simulink model "e5_3blocks_nn"  (R2020a)
settings: Solver=VariableStepAuto  StartTime=0.0  StopTime=10.0  RelTol=1e-3
undefined symbols (not defined in the file or in its folder): Quad
libraries: neural x123
(part 1 of 6)
settings Model: Creator=kekatos  LastModifiedBy=kekatos

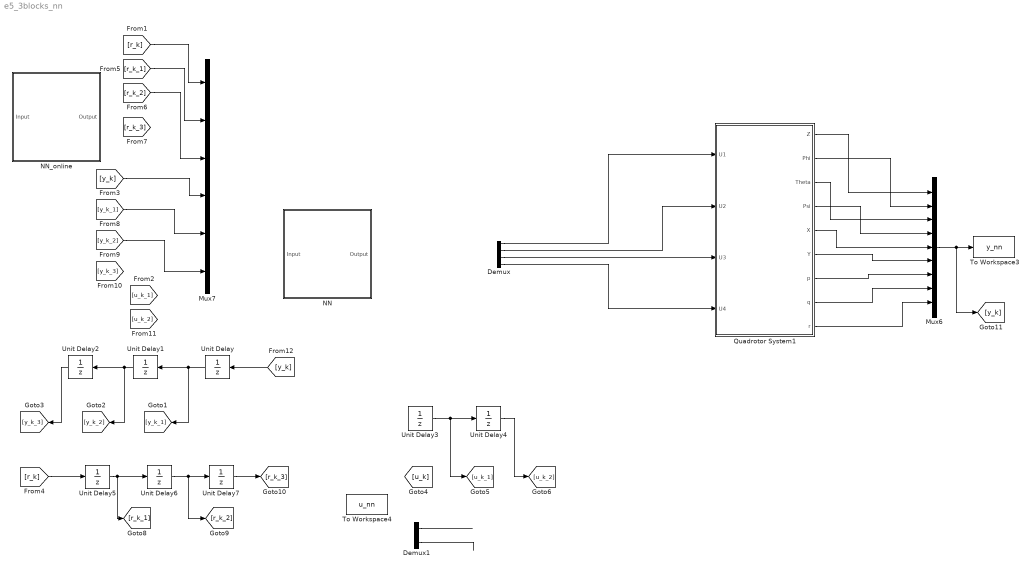
== system e5_3blocks_nn ==
  Demux : Demux
  Demux1 : Demux  Outputs=2
  Mux6 : Mux  Inputs=9
  Mux7 : Mux  Inputs=6
  NN : Subsystem
      mask help: Feed-Forward Neural Network
      mask Display: e = 0.06;c1 = [120 150 230]/255;c2 = ([120 150 230]+0)/383;c3 = ([120 150 230]+128)/383;patch([0 1 1 0],[0 0 1 1],c1);patch([0 1 1 1-e 1-e 0+e],[0 0 1 1-e 0+e 0+e],c2);patch([0 0 1 1-e 0+e 0+e],[0 1 1 1-e 1-e 0+e],c3);plot([0 1 1 0 0],[0 0 1 1 0]);fprintf('NNET');port_label('input',1,' Input');port_label('output',1,'Output ');
  NN_online : Subsystem
      mask help: Feed-Forward Neural Network
      mask Display: e = 0.06;c1 = [120 150 230]/255;c2 = ([120 150 230]+0)/383;c3 = ([120 150 230]+128)/383;patch([0 1 1 0],[0 0 1 1],c1);patch([0 1 1 1-e 1-e 0+e],[0 0 1 1-e 0+e 0+e],c2);patch([0 0 1 1-e 0+e 0+e],[0 1 1 1-e 1-e 0+e],c3);plot([0 1 1 0 0],[0 0 1 1 0]);fprintf('NNET');port_label('input',1,' Input');port_label('output',1,'Output ');
  Quadrotor System1 : Subsystem
  To Workspace3 : ToWorkspace  VariableName=y_nn  SaveFormat=Structure With Time  SampleTime=0.01
  To Workspace4 : ToWorkspace  VariableName=u_nn  SaveFormat=Structure With Time  SampleTime=0.01
  Unit Delay{,1..7} (8 alike) : UnitDelay  SampleTime=-1  HasFrameUpgradeWarning=on
  wires:
  Quadrotor System1/7(p) -> Mux6/7
  Unit Delay2/1 -> [y_k_3]
  Quadrotor System1/1(Z) -> Mux6/1
  [y_k] -> Unit Delay/1
  Unit Delay6/1 -> [r_k_2], Unit Delay7/1
  [r_k] -> Mux7/1
  Quadrotor System1/4(Psi) -> Mux6/4
  Unit Delay4/1 -> [u_k_2]
  Quadrotor System1/9(r) -> Mux6/9
  Unit Delay7/1 -> [r_k_3]
  Unit Delay1/1 -> Unit Delay2/1, [y_k_2]
  Unit Delay/1 -> Unit Delay1/1, [y_k_1]
  [r_k_2] -> Mux7/3
  Quadrotor System1/5(X) -> Mux6/5
  Demux/1 -> Quadrotor System1/1(U1)
  Mux6/1 -> [y_k], To Workspace3/1
  Unit Delay3/1 -> [u_k_1], Unit Delay4/1
  Quadrotor System1/3(Theta) -> Mux6/3
  Demux1/1 -> ?
  Quadrotor System1/8(q) -> Mux6/8
  [y_k] -> Mux7/4
  Demux/4 -> Quadrotor System1/4(U4)
  Quadrotor System1/2(Phi) -> Mux6/2
  Demux1/2 -> ?
  Quadrotor System1/6(Y) -> Mux6/6
  Demux/2 -> Quadrotor System1/2(U2)
  [y_k_2] -> Mux7/6
  [r_k_1] -> Mux7/2
  [y_k_1] -> Mux7/5
  Demux/3 -> Quadrotor System1/3(U3)
  [r_k] -> Unit Delay5/1
  Unit Delay5/1 -> [r_k_1], Unit Delay6/1

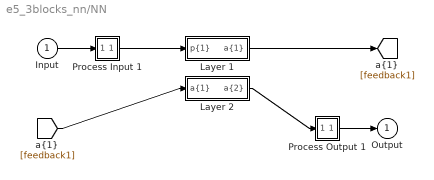
== system e5_3blocks_nn/NN ==
  Input : Inport  PortDimensions=15
      mask Display: e = 0.06;c1 = [120 230 180]/255;c2 = ([120 230 180]+0)/(256+128);c3 = ([120 230 180]+128)/(256+128);patch([0 1 1 0],[0 0 1 1],c1);patch([0 1 1 1-e 1-e 0+e],[0 0 1 1-e 0+e 0+e],c2);patch([0 0 1 1-e 0+e 0+e],[0 1 1 1-e 1-e 0+e],c3);plot([0 1 1 0 0],[0 0 1 1 0]);
  Layer 1 : Subsystem
      mask Display: e = 0.06;c1 = [120 150 230]/255;c2 = ([120 150 230]+0)/383;c3 = ([120 150 230]+128)/383;patch([0 1 1 0],[0 0 1 1],c1);patch([0 1 1 1-e 1-e 0+e],[0 0 1 1-e 0+e 0+e],c2);patch([0 0 1 1-e 0+e 0+e],[0 1 1 1-e 1-e 0+e],c3);plot([0 1 1 0 0],[0 0 1 1 0]);
  Layer 2 : Subsystem
      mask Display: e = 0.06;c1 = [120 150 230]/255;c2 = ([120 150 230]+0)/383;c3 = ([120 150 230]+128)/383;patch([0 1 1 0],[0 0 1 1],c1);patch([0 1 1 1-e 1-e 0+e],[0 0 1 1-e 0+e 0+e],c2);patch([0 0 1 1-e 0+e 0+e],[0 1 1 1-e 1-e 0+e],c3);plot([0 1 1 0 0],[0 0 1 1 0]);
  Process Input 1 : Subsystem
      mask Display: e = 0.06;c1 = [120 150 230]/255;c2 = ([120 150 230]+0)/383;c3 = ([120 150 230]+128)/383;patch([0 1 1 0],[0 0 1 1],c1);patch([0 1 1 1-e 1-e 0+e],[0 0 1 1-e 0+e 0+e],c2);patch([0 0 1 1-e 0+e 0+e],[0 1 1 1-e 1-e 0+e],c3);plot([0 1 1 0 0],[0 0 1 1 0]);
  Process Output 1 : Subsystem
      mask Display: e = 0.06;c1 = [120 150 230]/255;c2 = ([120 150 230]+0)/383;c3 = ([120 150 230]+128)/383;patch([0 1 1 0],[0 0 1 1],c1);patch([0 1 1 1-e 1-e 0+e],[0 0 1 1-e 0+e 0+e],c2);patch([0 0 1 1-e 0+e 0+e],[0 1 1 1-e 1-e 0+e],c3);plot([0 1 1 0 0],[0 0 1 1 0]);
  Output : Outport  InitialOutput=[0;0]
      mask Display: e = 0.06;c1 = [120 230 180]/255;c2 = ([120 230 180]+0)/(256+128);c3 = ([120 230 180]+128)/(256+128);patch([0 1 1 0],[0 0 1 1],c1);patch([0 1 1 1-e 1-e 0+e],[0 0 1 1-e 0+e 0+e],c2);patch([0 0 1 1-e 0+e 0+e],[0 1 1 1-e 1-e 0+e],c3);plot([0 1 1 0 0],[0 0 1 1 0]);
  wires:
  Input/1 -> Process Input 1/1(x)
  Process Output 1/1(y) -> Output/1
  Process Input 1/1(p) -> Layer 1/1("p{1}")
  Layer 1/1("a{1}") -> [feedback1]
  [feedback1] -> Layer 2/1("a{1} ")
  Layer 2/1("a{2}") -> Process Output 1/1(a)

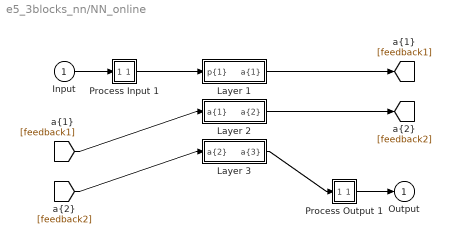
== system e5_3blocks_nn/NN_online ==
  Input : Inport  PortDimensions=20
      mask Display: e = 0.06;c1 = [120 230 180]/255;c2 = ([120 230 180]+0)/(256+128);c3 = ([120 230 180]+128)/(256+128);patch([0 1 1 0],[0 0 1 1],c1);patch([0 1 1 1-e 1-e 0+e],[0 0 1 1-e 0+e 0+e],c2);patch([0 0 1 1-e 0+e 0+e],[0 1 1 1-e 1-e 0+e],c3);plot([0 1 1 0 0],[0 0 1 1 0]);
  Layer 1 : Subsystem
      mask Display: e = 0.06;c1 = [120 150 230]/255;c2 = ([120 150 230]+0)/383;c3 = ([120 150 230]+128)/383;patch([0 1 1 0],[0 0 1 1],c1);patch([0 1 1 1-e 1-e 0+e],[0 0 1 1-e 0+e 0+e],c2);patch([0 0 1 1-e 0+e 0+e],[0 1 1 1-e 1-e 0+e],c3);plot([0 1 1 0 0],[0 0 1 1 0]);
  Layer 2 : Subsystem
      mask Display: e = 0.06;c1 = [120 150 230]/255;c2 = ([120 150 230]+0)/383;c3 = ([120 150 230]+128)/383;patch([0 1 1 0],[0 0 1 1],c1);patch([0 1 1 1-e 1-e 0+e],[0 0 1 1-e 0+e 0+e],c2);patch([0 0 1 1-e 0+e 0+e],[0 1 1 1-e 1-e 0+e],c3);plot([0 1 1 0 0],[0 0 1 1 0]);
  Layer 3 : Subsystem
      mask Display: e = 0.06;c1 = [120 150 230]/255;c2 = ([120 150 230]+0)/383;c3 = ([120 150 230]+128)/383;patch([0 1 1 0],[0 0 1 1],c1);patch([0 1 1 1-e 1-e 0+e],[0 0 1 1-e 0+e 0+e],c2);patch([0 0 1 1-e 0+e 0+e],[0 1 1 1-e 1-e 0+e],c3);plot([0 1 1 0 0],[0 0 1 1 0]);
  Process Input 1 : Subsystem
      mask Display: e = 0.06;c1 = [120 150 230]/255;c2 = ([120 150 230]+0)/383;c3 = ([120 150 230]+128)/383;patch([0 1 1 0],[0 0 1 1],c1);patch([0 1 1 1-e 1-e 0+e],[0 0 1 1-e 0+e 0+e],c2);patch([0 0 1 1-e 0+e 0+e],[0 1 1 1-e 1-e 0+e],c3);plot([0 1 1 0 0],[0 0 1 1 0]);
  Process Output 1 : Subsystem
      mask Display: e = 0.06;c1 = [120 150 230]/255;c2 = ([120 150 230]+0)/383;c3 = ([120 150 230]+128)/383;patch([0 1 1 0],[0 0 1 1],c1);patch([0 1 1 1-e 1-e 0+e],[0 0 1 1-e 0+e 0+e],c2);patch([0 0 1 1-e 0+e 0+e],[0 1 1 1-e 1-e 0+e],c3);plot([0 1 1 0 0],[0 0 1 1 0]);
  Output : Outport  InitialOutput=[0;0]
      mask Display: e = 0.06;c1 = [120 230 180]/255;c2 = ([120 230 180]+0)/(256+128);c3 = ([120 230 180]+128)/(256+128);patch([0 1 1 0],[0 0 1 1],c1);patch([0 1 1 1-e 1-e 0+e],[0 0 1 1-e 0+e 0+e],c2);patch([0 0 1 1-e 0+e 0+e],[0 1 1 1-e 1-e 0+e],c3);plot([0 1 1 0 0],[0 0 1 1 0]);
  wires:
  Input/1 -> Process Input 1/1(x)
  Process Output 1/1(y) -> Output/1
  Process Input 1/1(p) -> Layer 1/1("p{1}")
  Layer 1/1("a{1}") -> [feedback1]
  [feedback1] -> Layer 2/1("a{1} ")
  Layer 2/1("a{2}") -> [feedback2]
  [feedback2] -> Layer 3/1("a{2} ")
  Layer 3/1("a{3}") -> Process Output 1/1(a)

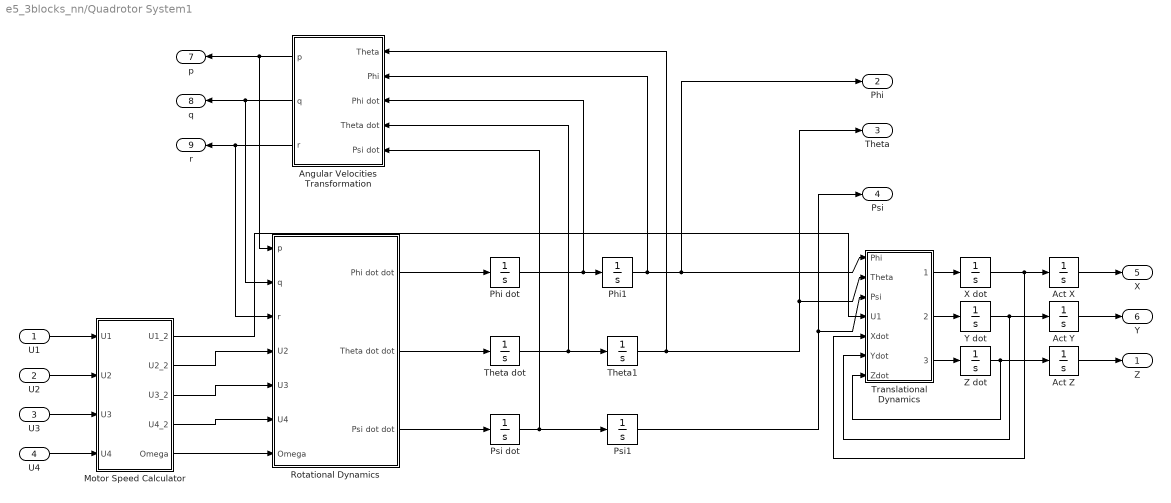
== system e5_3blocks_nn/Quadrotor System1 ==
  U1 : Inport
  U2 : Inport  Port=2
  U3 : Inport  Port=3
  U4 : Inport  Port=4
  Act X : Integrator
  Act Y : Integrator
  Act Z : Integrator
  Angular Velocities Transformation : Subsystem
  Motor Speed Calculator : Subsystem
  Phi dot : Integrator
  Phi1 : Integrator  ZeroCross=off
  Psi dot : Integrator  ZeroCross=off
  Psi1 : Integrator  ZeroCross=off
  Rotational Dynamics : Subsystem
  Theta dot : Integrator  ZeroCross=off
  Theta1 : Integrator  ZeroCross=off
  Translational Dynamics : Subsystem
  X dot : Integrator
  Y dot : Integrator
  Z dot : Integrator
  Z : Outport  VectorParamsAs1DForOutWhenUnconnected=off
  Phi : Outport  Port=2  VectorParamsAs1DForOutWhenUnconnected=off
  Theta : Outport  Port=3  VectorParamsAs1DForOutWhenUnconnected=off
  Psi : Outport  Port=4  VectorParamsAs1DForOutWhenUnconnected=off
  X : Outport  Port=5  VectorParamsAs1DForOutWhenUnconnected=off
  Y : Outport  Port=6  VectorParamsAs1DForOutWhenUnconnected=off
  p : Outport  Port=7  VectorParamsAs1DForOutWhenUnconnected=off
  q : Outport  Port=8  VectorParamsAs1DForOutWhenUnconnected=off
  r : Outport  Port=9  VectorParamsAs1DForOutWhenUnconnected=off
  wires:
  Rotational Dynamics/2(Theta dot dot) -> Theta dot/1
  Motor Speed Calculator/5(Omega) -> Rotational Dynamics/7(Omega)
  Phi1/1 -> Translational Dynamics/1(Phi), Phi/1, Angular Velocities Transformation/2(Phi)
  Theta1/1 -> Translational Dynamics/2(Theta), Theta/1, Angular Velocities Transformation/1(Theta)
  Psi1/1 -> Translational Dynamics/3(Psi), Psi/1
  Translational Dynamics/1(x dotdot) -> X dot/1
  X dot/1 -> Act X/1, Translational Dynamics/5(Xdot)
  Y dot/1 -> Act Y/1, Translational Dynamics/6(Ydot)
  Translational Dynamics/2(y dotdot) -> Y dot/1
  Z dot/1 -> Translational Dynamics/7(Zdot), Act Z/1
  Translational Dynamics/3(z dotdot) -> Z dot/1
  Act X/1 -> X/1
  Act Y/1 -> Y/1
  Act Z/1 -> Z/1
  Psi dot/1 -> Psi1/1, Angular Velocities Transformation/5(Psi dot)
  Theta dot/1 -> Theta1/1, Angular Velocities Transformation/4(Theta dot)
  Phi dot/1 -> Phi1/1, Angular Velocities Transformation/3(Phi dot)
  Rotational Dynamics/3(Psi dot dot) -> Psi dot/1
  Rotational Dynamics/1(Phi dot dot) -> Phi dot/1
  U4/1 -> Motor Speed Calculator/4(U4)
  U2/1 -> Motor Speed Calculator/2(U2)
  U3/1 -> Motor Speed Calculator/3(U3)
  Motor Speed Calculator/2(U2_2) -> Rotational Dynamics/4(U2)
  Motor Speed Calculator/3(U3_2) -> Rotational Dynamics/5(U3)
  Motor Speed Calculator/1(U1_2) -> Translational Dynamics/4(U1)
  Motor Speed Calculator/4(U4_2) -> Rotational Dynamics/6(U4)
  Angular Velocities Transformation/1(p) -> Rotational Dynamics/1(p), p/1
  Angular Velocities Transformation/2(q) -> Rotational Dynamics/2(q), q/1
  Angular Velocities Transformation/3(r) -> Rotational Dynamics/3(r), r/1
  U1/1 -> Motor Speed Calculator/1(U1)

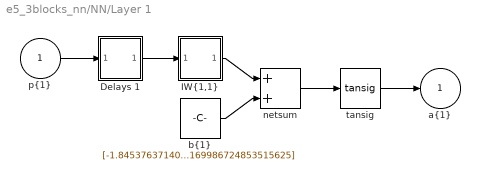
== system e5_3blocks_nn/NN/Layer 1 ==
  "p{1}" : Inport  PortDimensions=15
      mask Display: e = 0.06;c1 = [120 230 180]/255;c2 = ([120 230 180]+0)/(256+128);c3 = ([120 230 180]+128)/(256+128);patch([0 1 1 0],[0 0 1 1],c1);patch([0 1 1 1-e 1-e 0+e],[0 0 1 1-e 0+e 0+e],c2);patch([0 0 1 1-e 0+e 0+e],[0 1 1 1-e 1-e 0+e],c3);plot([0 1 1 0 0],[0 0 1 1 0]);
  Delays 1 : Subsystem
      mask Display: e = 0.06;c1 = [120 150 230]/255;c2 = ([120 150 230]+0)/383;c3 = ([120 150 230]+128)/383;patch([0 1 1 0],[0 0 1 1],c1);patch([0 1 1 1-e 1-e 0+e],[0 0 1 1-e 0+e 0+e],c2);patch([0 0 1 1-e 0+e 0+e],[0 1 1 1-e 1-e 0+e],c3);plot([0 1 1 0 0],[0 0 1 1 0]);disp('0');
  "IW{1,1}" : Subsystem
      mask Display: e = 0.06;c1 = [120 150 230]/255;c2 = ([120 150 230]+0)/383;c3 = ([120 150 230]+128)/383;patch([0 1 1 0],[0 0 1 1],c1);patch([0 1 1 1-e 1-e 0+e],[0 0 1 1-e 0+e 0+e],c2);patch([0 0 1 1-e 0+e 0+e],[0 1 1 1-e 1-e 0+e],c3);plot([0 1 1 0 0],[0 0 1 1 0]);disp('W');
  "b{1}" : Constant  Value=[-1.84537637140731280993577456683851778507232666015625;-1.7532825244992047419856362466816790401935577392578125;1.71407838156578673505237020435743033885955810546875;-1.6342052333083547654979383878526277840137481689453125;-1.5438537489742396591196893496089614927768707275390625;1.4283080018807214894849266784149222075939178466796875;-1.404821018307291780047307838685810565948486328125;1.287885767879537457503147379611618816852569580078125;1.25502611674529962471069666207768023014068603515625;1.0972360429977421336644738403265364468097686767578125;1.131430962279293073180497231078334152698516845703125;-0.9955530066140656497708505412447266280651092529296875;-0.89412837469389450095746951774344779551029205322265625;0.85010871782267416474354604360996745526790618896484375;-0.80545016544390790613761055283248424530029296875;-0.70922638754411959638446205644868314266204833984375;-0.63105719893839429257553774732514284551143646240234375;-0.569988447775239048809226005687378346920013427734375;0.477593047053590902262243389486684463918209075927734375;0.403175590821758189630230617694905959069728851318359375;0.358673720801043760531001680647023022174835205078125;-0.2482304075266782150688271713079302571713924407958984375;0.15068110824116487389545682162861339747905731201171875;-0.1602803495511306020038233555169426836073398590087890625;-0.0987868360797714839538485875891637988388538360595703125;0.04171171965434290751506551941929501481354236602783203125;0.0939112815207025775077198659346322529017925262451171875;-0.177186006071735346889539641779265366494655609130859375;0.2396368639811528866712109220316051505506038665771484375;0.342981184701568242445546275121159851551055908203125;0.416928111920932209510937127561192028224468231201171875;-0.495950560740119616998100582350161857903003692626953125;-0.590456977511941705216713671688921749591827392578125;-0.6649151320152437705246484256349503993988037109375;-0.608626845880423150703109058667905628681182861328125;0.79801769557657376008563687719288282096385955810546875;0.89966865010810692648846043084631673991680145263671875;0.9564815597009614922541231862851418554782867431640625;-1.04442351552266732284124373109079897403717041015625;-1.0713399950107189706471899626194499433040618896484375;-1.191236975152814903111675448599271476268768310546875;-1.1699716443134151599991810144274495542049407958984375;-1.29708105375885995869111866340972483158111572265625;1.3771740284091971151525513050728477537631988525390625;1.3780962923269959308214538395986892282962799072265625;1.53107763486454206969256119919009506702423095703125;-1.625607738312811800795998351532034575939178466796875;-1.698033535260649262710330731351859867572784423828125;-1.740593156442128641714361947379074990749359130859375;-1.7825772239617221348595421659410931169986724853515625]
      mask Display: e = 0.06;c1 = [120 150 230]/255;c2 = ([120 150 230]+0)/383;c3 = ([120 150 230]+128)/383;patch([0 1 1 0],[0 0 1 1],c1);patch([0 1 1 1-e 1-e 0+e],[0 0 1 1-e 0+e 0+e],c2);patch([0 0 1 1-e 0+e 0+e],[0 1 1 1-e 1-e 0+e],c3);plot([0 1 1 0 0],[0 0 1 1 0]);disp('b');
  netsum : Sum  Inputs=2  InputSameDT=on  SaturateOnIntegerOverflow=on  OutDataTypeStr=Inherit: Same as first input
      mask Display: e = 0.06;c1 = [120 150 230]/255;c2 = ([120 150 230]+0)/383;c3 = ([120 150 230]+128)/383;patch([0 1 1 0],[0 0 1 1],c1);patch([0 1 1 1-e 1-e 0+e],[0 0 1 1-e 0+e 0+e],c2);patch([0 0 1 1-e 0+e 0+e],[0 1 1 1-e 1-e 0+e],c3);plot([0 1 1 0 0],[0 0 1 1 0]);disp('+');
  tansig : neural/Transfer Functions/tansig
  "a{1}" : Outport  InitialOutput=[0;0;0;0;0;0;0;0;0;0;0;0;0;0;0;0;0;0;0;0;0;0;0;0;0;0;0;0;0;0;0;0;0;0;0;0;0;0;0;0;0;0;0;0;0;0;0;0;0;0]
      mask Display: e = 0.06;c1 = [120 230 180]/255;c2 = ([120 230 180]+0)/(256+128);c3 = ([120 230 180]+128)/(256+128);patch([0 1 1 0],[0 0 1 1],c1);patch([0 1 1 1-e 1-e 0+e],[0 0 1 1-e 0+e 0+e],c2);patch([0 0 1 1-e 0+e 0+e],[0 1 1 1-e 1-e 0+e],c3);plot([0 1 1 0 0],[0 0 1 1 0]);
  wires:
  "p{1}"/1 -> Delays 1/1("p{1}")
  Delays 1/1("pd{1,1}") -> "IW{1,1}"/1("pd{1,1}")
  "IW{1,1}"/1("iz{1,1}") -> netsum/1
  "b{1}"/1 -> netsum/2
  netsum/1 -> tansig/1
  tansig/1 -> "a{1}"/1

== system e5_3blocks_nn/NN/Layer 2 ==
  "a{1} " : Inport  PortDimensions=50
      mask Display: e = 0.06;c1 = [120 230 180]/255;c2 = ([120 230 180]+0)/(256+128);c3 = ([120 230 180]+128)/(256+128);patch([0 1 1 0],[0 0 1 1],c1);patch([0 1 1 1-e 1-e 0+e],[0 0 1 1-e 0+e 0+e],c2);patch([0 0 1 1-e 0+e 0+e],[0 1 1 1-e 1-e 0+e],c3);plot([0 1 1 0 0],[0 0 1 1 0]);
  Delays 1 : Subsystem
      mask Display: e = 0.06;c1 = [120 150 230]/255;c2 = ([120 150 230]+0)/383;c3 = ([120 150 230]+128)/383;patch([0 1 1 0],[0 0 1 1],c1);patch([0 1 1 1-e 1-e 0+e],[0 0 1 1-e 0+e 0+e],c2);patch([0 0 1 1-e 0+e 0+e],[0 1 1 1-e 1-e 0+e],c3);plot([0 1 1 0 0],[0 0 1 1 0]);disp('0');
  "LW{2,1}" : Subsystem
      mask Display: e = 0.06;c1 = [120 150 230]/255;c2 = ([120 150 230]+0)/383;c3 = ([120 150 230]+128)/383;patch([0 1 1 0],[0 0 1 1],c1);patch([0 1 1 1-e 1-e 0+e],[0 0 1 1-e 0+e 0+e],c2);patch([0 0 1 1-e 0+e 0+e],[0 1 1 1-e 1-e 0+e],c3);plot([0 1 1 0 0],[0 0 1 1 0]);disp('W');
  "b{2}" : Constant  Value=[1.28161781860947154854102336685173213481903076171875;1.24192246401782568909766268916428089141845703125]
      mask Display: e = 0.06;c1 = [120 150 230]/255;c2 = ([120 150 230]+0)/383;c3 = ([120 150 230]+128)/383;patch([0 1 1 0],[0 0 1 1],c1);patch([0 1 1 1-e 1-e 0+e],[0 0 1 1-e 0+e 0+e],c2);patch([0 0 1 1-e 0+e 0+e],[0 1 1 1-e 1-e 0+e],c3);plot([0 1 1 0 0],[0 0 1 1 0]);disp('b');
  netsum : Sum  Inputs=2  InputSameDT=on  SaturateOnIntegerOverflow=on  OutDataTypeStr=Inherit: Same as first input
      mask Display: e = 0.06;c1 = [120 150 230]/255;c2 = ([120 150 230]+0)/383;c3 = ([120 150 230]+128)/383;patch([0 1 1 0],[0 0 1 1],c1);patch([0 1 1 1-e 1-e 0+e],[0 0 1 1-e 0+e 0+e],c2);patch([0 0 1 1-e 0+e 0+e],[0 1 1 1-e 1-e 0+e],c3);plot([0 1 1 0 0],[0 0 1 1 0]);disp('+');
  tansig : neural/Transfer Functions/tansig
  "a{2}" : Outport  InitialOutput=[0;0]
      mask Display: e = 0.06;c1 = [120 230 180]/255;c2 = ([120 230 180]+0)/(256+128);c3 = ([120 230 180]+128)/(256+128);patch([0 1 1 0],[0 0 1 1],c1);patch([0 1 1 1-e 1-e 0+e],[0 0 1 1-e 0+e 0+e],c2);patch([0 0 1 1-e 0+e 0+e],[0 1 1 1-e 1-e 0+e],c3);plot([0 1 1 0 0],[0 0 1 1 0]);
  wires:
  "a{1} "/1 -> Delays 1/1("p{2}")
  Delays 1/1("pd{2,1}") -> "LW{2,1}"/1("ad{2,1}")
  "LW{2,1}"/1("lz{2,1}") -> netsum/1
  "b{2}"/1 -> netsum/2
  netsum/1 -> tansig/1
  tansig/1 -> "a{2}"/1

== system e5_3blocks_nn/NN/Process Input 1 ==
  x : Inport  PortDimensions=15
      mask Display: e = 0.06;c1 = [120 230 180]/255;c2 = ([120 230 180]+0)/(256+128);c3 = ([120 230 180]+128)/(256+128);patch([0 1 1 0],[0 0 1 1],c1);patch([0 1 1 1-e 1-e 0+e],[0 0 1 1-e 0+e 0+e],c2);patch([0 0 1 1-e 0+e 0+e],[0 1 1 1-e 1-e 0+e],c3);plot([0 1 1 0 0],[0 0 1 1 0]);
  mapminmax : neural/Processing Functions/mapminmax  xmin=[3.43124452034659910282243799884e-05;0.000861098109347690978017386687071;0;0;0;0;-7.7003185079193718675164004317e-05;0;-0.0177130156218504447585004868415;-7.7003185079193718675164004317e-05;0;-0.0177130156218504447585004868415;-7.7003185079193718675164004317e-05;0;-0.0177130156218504447585004868415]  xmax=[0.290478472715819224791999886293;0.299196855135444139683897901705;0.290478472715819224791999886293;0.299196855135444139683897901705;0.290478472715819224791999886293;0.299196855135444139683897901705;8.37153844184080562487379473247e-05;0.341964637358954937074173585643;0.337708363299572378313229137348;8.37153844184080562487379473247e-05;0.341964637358954937074173585643;0.337708363299572378313229137348;8.37153844184080562487379473247e-05;0.341964637358954937074173585643;0.337708363299572378313229137348]  ymin=-1  ymax=1
  p : Outport  PortDimensions=15
      mask Display: e = 0.06;c1 = [120 230 180]/255;c2 = ([120 230 180]+0)/(256+128);c3 = ([120 230 180]+128)/(256+128);patch([0 1 1 0],[0 0 1 1],c1);patch([0 1 1 1-e 1-e 0+e],[0 0 1 1-e 0+e 0+e],c2);patch([0 0 1 1-e 0+e 0+e],[0 1 1 1-e 1-e 0+e],c3);plot([0 1 1 0 0],[0 0 1 1 0]);
  wires:
  x/1 -> mapminmax/1
  mapminmax/1 -> p/1

== system e5_3blocks_nn/NN/Process Output 1 ==
  a : Inport  PortDimensions=2
      mask Display: e = 0.06;c1 = [120 230 180]/255;c2 = ([120 230 180]+0)/(256+128);c3 = ([120 230 180]+128)/(256+128);patch([0 1 1 0],[0 0 1 1],c1);patch([0 1 1 1-e 1-e 0+e],[0 0 1 1-e 0+e 0+e],c2);patch([0 0 1 1-e 0+e 0+e],[0 1 1 1-e 1-e 0+e],c3);plot([0 1 1 0 0],[0 0 1 1 0]);
  mapminmax_reverse : neural/Processing Functions/mapminmax_reverse  xmin=[-0.0290478472715819252547575501922;-0.0225523089146122887593826078501]  xmax=[0.0181937723673191685536121298128;0.0299196855135444167439473517334]  ymin=-1  ymax=1
  y : Outport  PortDimensions=2
      mask Display: e = 0.06;c1 = [120 230 180]/255;c2 = ([120 230 180]+0)/(256+128);c3 = ([120 230 180]+128)/(256+128);patch([0 1 1 0],[0 0 1 1],c1);patch([0 1 1 1-e 1-e 0+e],[0 0 1 1-e 0+e 0+e],c2);patch([0 0 1 1-e 0+e 0+e],[0 1 1 1-e 1-e 0+e],c3);plot([0 1 1 0 0],[0 0 1 1 0]);
  wires:
  a/1 -> mapminmax_reverse/1
  mapminmax_reverse/1 -> y/1

== system e5_3blocks_nn/NN_online/Layer 1 ==
  "p{1}" : Inport  PortDimensions=20
      mask Display: e = 0.06;c1 = [120 230 180]/255;c2 = ([120 230 180]+0)/(256+128);c3 = ([120 230 180]+128)/(256+128);patch([0 1 1 0],[0 0 1 1],c1);patch([0 1 1 1-e 1-e 0+e],[0 0 1 1-e 0+e 0+e],c2);patch([0 0 1 1-e 0+e 0+e],[0 1 1 1-e 1-e 0+e],c3);plot([0 1 1 0 0],[0 0 1 1 0]);
  Delays 1 : Subsystem
      mask Display: e = 0.06;c1 = [120 150 230]/255;c2 = ([120 150 230]+0)/383;c3 = ([120 150 230]+128)/383;patch([0 1 1 0],[0 0 1 1],c1);patch([0 1 1 1-e 1-e 0+e],[0 0 1 1-e 0+e 0+e],c2);patch([0 0 1 1-e 0+e 0+e],[0 1 1 1-e 1-e 0+e],c3);plot([0 1 1 0 0],[0 0 1 1 0]);disp('0');
  "IW{1,1}" : Subsystem
      mask Display: e = 0.06;c1 = [120 150 230]/255;c2 = ([120 150 230]+0)/383;c3 = ([120 150 230]+128)/383;patch([0 1 1 0],[0 0 1 1],c1);patch([0 1 1 1-e 1-e 0+e],[0 0 1 1-e 0+e 0+e],c2);patch([0 0 1 1-e 0+e 0+e],[0 1 1 1-e 1-e 0+e],c3);plot([0 1 1 0 0],[0 0 1 1 0]);disp('W');
  "b{1}" : Constant  Value=[1.773843019974727486243182283942587673664093017578125;1.622878773289350373687511819298379123210906982421875;1.4561444625262309759960999144823290407657623291015625;1.381780857734258294300389025011099874973297119140625;-1.2744257887490910707839475435321219265460968017578125;1.2704629812613379424846016263472847640514373779296875;-0.94544009091574476855157627142034471035003662109375;-0.9337379344929856994639294498483650386333465576171875;-0.56109092582451458586234593894914723932743072509765625;-0.499047995113156950264254874127800576388835906982421875;-0.309368061599387844662345514734624885022640228271484375;0.3059387609359534021535864667384885251522064208984375;0.30987174868634070890038856305181980133056640625;-0.1240530062472051386901483738256501965224742889404296875;-0.2292650903033664200325603133023832924664020538330078125;0.1919116845205318389044890636796480976045131683349609375;-0.2367090426730429353341378373443149030208587646484375;0.632733666045173226422093648579902946949005126953125;-0.2539514671290665770442274151719175279140472412109375;0.273149558210549814329937134971260093152523040771484375;0.6098064760409156459530777283362112939357757568359375;-0.6655571849606707335311739370808936655521392822265625;-1.30952134522071705902135363430716097354888916015625;-1.124358574038685443241547545767389237880706787109375;-0.88408684534701631463349258410744369029998779296875;-1.070131743479656893924811811302788555622100830078125;-0.888301098263443833502606139518320560455322265625;1.60637678577253861789131406112574040889739990234375;-1.438485442130331914967200646060518920421600341796875;1.4975028639498424443132762462482787668704986572265625]
      mask Display: e = 0.06;c1 = [120 150 230]/255;c2 = ([120 150 230]+0)/383;c3 = ([120 150 230]+128)/383;patch([0 1 1 0],[0 0 1 1],c1);patch([0 1 1 1-e 1-e 0+e],[0 0 1 1-e 0+e 0+e],c2);patch([0 0 1 1-e 0+e 0+e],[0 1 1 1-e 1-e 0+e],c3);plot([0 1 1 0 0],[0 0 1 1 0]);disp('b');
  netsum : Sum  Inputs=2  InputSameDT=on  SaturateOnIntegerOverflow=on  OutDataTypeStr=Inherit: Same as first input
      mask Display: e = 0.06;c1 = [120 150 230]/255;c2 = ([120 150 230]+0)/383;c3 = ([120 150 230]+128)/383;patch([0 1 1 0],[0 0 1 1],c1);patch([0 1 1 1-e 1-e 0+e],[0 0 1 1-e 0+e 0+e],c2);patch([0 0 1 1-e 0+e 0+e],[0 1 1 1-e 1-e 0+e],c3);plot([0 1 1 0 0],[0 0 1 1 0]);disp('+');
  tansig : neural/Transfer Functions/tansig
  "a{1}" : Outport  InitialOutput=[0;0;0;0;0;0;0;0;0;0;0;0;0;0;0;0;0;0;0;0;0;0;0;0;0;0;0;0;0;0]
      mask Display: e = 0.06;c1 = [120 230 180]/255;c2 = ([120 230 180]+0)/(256+128);c3 = ([120 230 180]+128)/(256+128);patch([0 1 1 0],[0 0 1 1],c1);patch([0 1 1 1-e 1-e 0+e],[0 0 1 1-e 0+e 0+e],c2);patch([0 0 1 1-e 0+e 0+e],[0 1 1 1-e 1-e 0+e],c3);plot([0 1 1 0 0],[0 0 1 1 0]);
  wires:
  "p{1}"/1 -> Delays 1/1("p{1}")
  Delays 1/1("pd{1,1}") -> "IW{1,1}"/1("pd{1,1}")
  "IW{1,1}"/1("iz{1,1}") -> netsum/1
  "b{1}"/1 -> netsum/2
  netsum/1 -> tansig/1
  tansig/1 -> "a{1}"/1

== system e5_3blocks_nn/NN_online/Layer 2 ==
  "a{1} " : Inport  PortDimensions=30
      mask Display: e = 0.06;c1 = [120 230 180]/255;c2 = ([120 230 180]+0)/(256+128);c3 = ([120 230 180]+128)/(256+128);patch([0 1 1 0],[0 0 1 1],c1);patch([0 1 1 1-e 1-e 0+e],[0 0 1 1-e 0+e 0+e],c2);patch([0 0 1 1-e 0+e 0+e],[0 1 1 1-e 1-e 0+e],c3);plot([0 1 1 0 0],[0 0 1 1 0]);
  Delays 1 : Subsystem
      mask Display: e = 0.06;c1 = [120 150 230]/255;c2 = ([120 150 230]+0)/383;c3 = ([120 150 230]+128)/383;patch([0 1 1 0],[0 0 1 1],c1);patch([0 1 1 1-e 1-e 0+e],[0 0 1 1-e 0+e 0+e],c2);patch([0 0 1 1-e 0+e 0+e],[0 1 1 1-e 1-e 0+e],c3);plot([0 1 1 0 0],[0 0 1 1 0]);disp('0');
  "LW{2,1}" : Subsystem
      mask Display: e = 0.06;c1 = [120 150 230]/255;c2 = ([120 150 230]+0)/383;c3 = ([120 150 230]+128)/383;patch([0 1 1 0],[0 0 1 1],c1);patch([0 1 1 1-e 1-e 0+e],[0 0 1 1-e 0+e 0+e],c2);patch([0 0 1 1-e 0+e 0+e],[0 1 1 1-e 1-e 0+e],c3);plot([0 1 1 0 0],[0 0 1 1 0]);disp('W');
  "b{2}" : Constant  Value=[-1.6104661092221810303470874714548699557781219482421875;1.5232595697190998151882013189606368541717529296875;-1.2985182846392240296751197092817164957523345947265625;1.204590044376149027272049352177418768405914306640625;1.251678863338696157114782181452028453350067138671875;1.01494224022407575347415331634692847728729248046875;-0.96543772869886701482045054945047013461589813232421875;0.8031921754411264213757704055751673877239227294921875;0.6568352782723023697286635069758631289005279541015625;-0.6066769298996559367509462390444241464138031005859375;-0.440273855967682259393569665917311795055866241455078125;-0.457113530252571009793172152058104984462261199951171875;0.3196333899809051803941883918014355003833770751953125;0.06259764700825420913332663985784165561199188232421875;-0.11598172235965320542305789786041714251041412353515625;0.08490411563825796259497025175733142532408237457275390625;-0.1396995888852784195588441207291907630860805511474609375;0.389117868210294926001324711251072585582733154296875;0.3804331308467254757488262839615345001220703125;0.432664243991749242201905190086108632385730743408203125;0.64662355869928178631056425729184411466121673583984375;0.70856996620086010185701752561726607382297515869140625;0.64040526260070895769871412994689308106899261474609375;-0.8350820789884731976115972429397515952587127685546875;-0.997827373290781860504239375586621463298797607421875;-1.17393533527395543814009215566329658031463623046875;-1.241355747799975706158193133887834846973419189453125;-1.3013259212684278320892872216063551604747772216796875;-1.4307958545471184397257502496358938515186309814453125;-1.5442056771441412532652748268446885049343109130859375]
      mask Display: e = 0.06;c1 = [120 150 230]/255;c2 = ([120 150 230]+0)/383;c3 = ([120 150 230]+128)/383;patch([0 1 1 0],[0 0 1 1],c1);patch([0 1 1 1-e 1-e 0+e],[0 0 1 1-e 0+e 0+e],c2);patch([0 0 1 1-e 0+e 0+e],[0 1 1 1-e 1-e 0+e],c3);plot([0 1 1 0 0],[0 0 1 1 0]);disp('b');
  netsum : Sum  Inputs=2  InputSameDT=on  SaturateOnIntegerOverflow=on  OutDataTypeStr=Inherit: Same as first input
      mask Display: e = 0.06;c1 = [120 150 230]/255;c2 = ([120 150 230]+0)/383;c3 = ([120 150 230]+128)/383;patch([0 1 1 0],[0 0 1 1],c1);patch([0 1 1 1-e 1-e 0+e],[0 0 1 1-e 0+e 0+e],c2);patch([0 0 1 1-e 0+e 0+e],[0 1 1 1-e 1-e 0+e],c3);plot([0 1 1 0 0],[0 0 1 1 0]);disp('+');
  tansig : neural/Transfer Functions/tansig
  "a{2}" : Outport  InitialOutput=[0;0;0;0;0;0;0;0;0;0;0;0;0;0;0;0;0;0;0;0;0;0;0;0;0;0;0;0;0;0]
      mask Display: e = 0.06;c1 = [120 230 180]/255;c2 = ([120 230 180]+0)/(256+128);c3 = ([120 230 180]+128)/(256+128);patch([0 1 1 0],[0 0 1 1],c1);patch([0 1 1 1-e 1-e 0+e],[0 0 1 1-e 0+e 0+e],c2);patch([0 0 1 1-e 0+e 0+e],[0 1 1 1-e 1-e 0+e],c3);plot([0 1 1 0 0],[0 0 1 1 0]);
  wires:
  "a{1} "/1 -> Delays 1/1("p{2}")
  Delays 1/1("pd{2,1}") -> "LW{2,1}"/1("ad{2,1}")
  "LW{2,1}"/1("lz{2,1}") -> netsum/1
  "b{2}"/1 -> netsum/2
  netsum/1 -> tansig/1
  tansig/1 -> "a{2}"/1

== system e5_3blocks_nn/NN_online/Layer 3 ==
  "a{2} " : Inport  PortDimensions=30
      mask Display: e = 0.06;c1 = [120 230 180]/255;c2 = ([120 230 180]+0)/(256+128);c3 = ([120 230 180]+128)/(256+128);patch([0 1 1 0],[0 0 1 1],c1);patch([0 1 1 1-e 1-e 0+e],[0 0 1 1-e 0+e 0+e],c2);patch([0 0 1 1-e 0+e 0+e],[0 1 1 1-e 1-e 0+e],c3);plot([0 1 1 0 0],[0 0 1 1 0]);
  Delays 1 : Subsystem
      mask Display: e = 0.06;c1 = [120 150 230]/255;c2 = ([120 150 230]+0)/383;c3 = ([120 150 230]+128)/383;patch([0 1 1 0],[0 0 1 1],c1);patch([0 1 1 1-e 1-e 0+e],[0 0 1 1-e 0+e 0+e],c2);patch([0 0 1 1-e 0+e 0+e],[0 1 1 1-e 1-e 0+e],c3);plot([0 1 1 0 0],[0 0 1 1 0]);disp('0');
  "LW{3,2}" : Subsystem
      mask Display: e = 0.06;c1 = [120 150 230]/255;c2 = ([120 150 230]+0)/383;c3 = ([120 150 230]+128)/383;patch([0 1 1 0],[0 0 1 1],c1);patch([0 1 1 1-e 1-e 0+e],[0 0 1 1-e 0+e 0+e],c2);patch([0 0 1 1-e 0+e 0+e],[0 1 1 1-e 1-e 0+e],c3);plot([0 1 1 0 0],[0 0 1 1 0]);disp('W');
  "b{3}" : Constant  Value=[-0.38962628052624814767312955154920928180217742919921875;0.76841817652397181870327358410577289760112762451171875]
      mask Display: e = 0.06;c1 = [120 150 230]/255;c2 = ([120 150 230]+0)/383;c3 = ([120 150 230]+128)/383;patch([0 1 1 0],[0 0 1 1],c1);patch([0 1 1 1-e 1-e 0+e],[0 0 1 1-e 0+e 0+e],c2);patch([0 0 1 1-e 0+e 0+e],[0 1 1 1-e 1-e 0+e],c3);plot([0 1 1 0 0],[0 0 1 1 0]);disp('b');
  netsum : Sum  Inputs=2  InputSameDT=on  SaturateOnIntegerOverflow=on  OutDataTypeStr=Inherit: Same as first input
      mask Display: e = 0.06;c1 = [120 150 230]/255;c2 = ([120 150 230]+0)/383;c3 = ([120 150 230]+128)/383;patch([0 1 1 0],[0 0 1 1],c1);patch([0 1 1 1-e 1-e 0+e],[0 0 1 1-e 0+e 0+e],c2);patch([0 0 1 1-e 0+e 0+e],[0 1 1 1-e 1-e 0+e],c3);plot([0 1 1 0 0],[0 0 1 1 0]);disp('+');
  purelin : neural/Transfer Functions/purelin
  "a{3}" : Outport  InitialOutput=[0;0]
      mask Display: e = 0.06;c1 = [120 230 180]/255;c2 = ([120 230 180]+0)/(256+128);c3 = ([120 230 180]+128)/(256+128);patch([0 1 1 0],[0 0 1 1],c1);patch([0 1 1 1-e 1-e 0+e],[0 0 1 1-e 0+e 0+e],c2);patch([0 0 1 1-e 0+e 0+e],[0 1 1 1-e 1-e 0+e],c3);plot([0 1 1 0 0],[0 0 1 1 0]);
  wires:
  "a{2} "/1 -> Delays 1/1("p{3}")
  Delays 1/1("pd{3,2}") -> "LW{3,2}"/1("ad{3,2}")
  "LW{3,2}"/1("lz{3,2}") -> netsum/1
  "b{3}"/1 -> netsum/2
  netsum/1 -> purelin/1
  purelin/1 -> "a{3}"/1

== system e5_3blocks_nn/NN_online/Process Input 1 ==
  x : Inport  PortDimensions=20
      mask Display: e = 0.06;c1 = [120 230 180]/255;c2 = ([120 230 180]+0)/(256+128);c3 = ([120 230 180]+128)/(256+128);patch([0 1 1 0],[0 0 1 1],c1);patch([0 1 1 1-e 1-e 0+e],[0 0 1 1-e 0+e 0+e],c2);patch([0 0 1 1-e 0+e 0+e],[0 1 1 1-e 1-e 0+e],c3);plot([0 1 1 0 0],[0 0 1 1 0]);
  mapminmax : neural/Processing Functions/mapminmax  xmin=[0.206250000000000072164496600635;0.000591715976331361062992564292529;0;0;0;0;0;0;-1.24286750523964959456741513621e-05;0;-0.0107075553863898928486086958856;-1.24286750523964959456741513621e-05;0;-0.0107075553863898928486086958856;-1.24286750523964959456741513621e-05;0;-0.0107075553863898928486086958856;-1.24286750523964959456741513621e-05;0;-0.0107075553863898928486086958856]  xmax=[0.387500000000000011102230246252;0.0923076923076923128164139598084;0.387500000000000011102230246252;0.0923076923076923128164139598084;0.387500000000000011102230246252;0.0923076923076923128164139598084;0.387500000000000011102230246252;0.0923076923076923128164139598084;5.35078896628240365906763187365e-05;0.453428937371301687964120219476;0.100496355467121947779851609539;5.35078896628240365906763187365e-05;0.453428937371301687964120219476;0.100496355467121947779851609539;5.35078896628240365906763187365e-05;0.453428937371301687964120219476;0.100496355467121947779851609539;5.35078896628240365906763187365e-05;0.453428937371301687964120219476;0.100496355467121947779851609539]  ymin=-1  ymax=1
  p : Outport  PortDimensions=20
      mask Display: e = 0.06;c1 = [120 230 180]/255;c2 = ([120 230 180]+0)/(256+128);c3 = ([120 230 180]+128)/(256+128);patch([0 1 1 0],[0 0 1 1],c1);patch([0 1 1 1-e 1-e 0+e],[0 0 1 1-e 0+e 0+e],c2);patch([0 0 1 1-e 0+e 0+e],[0 1 1 1-e 1-e 0+e],c3);plot([0 1 1 0 0],[0 0 1 1 0]);
  wires:
  x/1 -> mapminmax/1
  mapminmax/1 -> p/1

== system e5_3blocks_nn/NN_online/Process Output 1 ==
  a : Inport  PortDimensions=2
      mask Display: e = 0.06;c1 = [120 230 180]/255;c2 = ([120 230 180]+0)/(256+128);c3 = ([120 230 180]+128)/(256+128);patch([0 1 1 0],[0 0 1 1],c1);patch([0 1 1 1-e 1-e 0+e],[0 0 1 1-e 0+e 0+e],c2);patch([0 0 1 1-e 0+e 0+e],[0 1 1 1-e 1-e 0+e],c3);plot([0 1 1 0 0],[0 0 1 1 0]);
  mapminmax_reverse : neural/Processing Functions/mapminmax_reverse  xmin=[-0.0387500000000000066613381477509;-0.00873707378433970748010661822036]  xmax=[0.0165451992159274009763780810545;0.00897959183673469572839476171566]  ymin=-1  ymax=1
  y : Outport  PortDimensions=2
      mask Display: e = 0.06;c1 = [120 230 180]/255;c2 = ([120 230 180]+0)/(256+128);c3 = ([120 230 180]+128)/(256+128);patch([0 1 1 0],[0 0 1 1],c1);patch([0 1 1 1-e 1-e 0+e],[0 0 1 1-e 0+e 0+e],c2);patch([0 0 1 1-e 0+e 0+e],[0 1 1 1-e 1-e 0+e],c3);plot([0 1 1 0 0],[0 0 1 1 0]);
  wires:
  a/1 -> mapminmax_reverse/1
  mapminmax_reverse/1 -> y/1

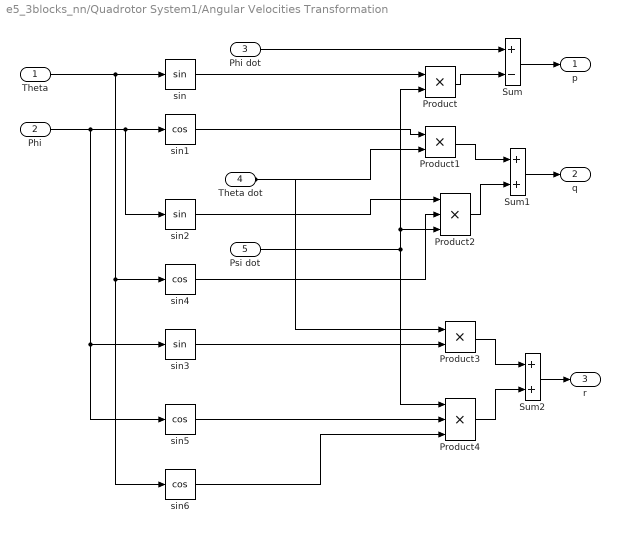
== system e5_3blocks_nn/Quadrotor System1/Angular Velocities Transformation ==
  Theta : Inport
  Phi : Inport  Port=2
  Phi dot : Inport  Port=3
  Theta dot : Inport  Port=4
  Psi dot : Inport  Port=5
  Product : Product  RndMeth=Zero
  Product1 : Product  RndMeth=Zero
  Product2 : Product  Inputs=3  RndMeth=Zero
  Product3 : Product  RndMeth=Zero
  Product4 : Product  Inputs=3  RndMeth=Zero
  Sum : Sum  Inputs=+-
  Sum1 : Sum
  Sum2 : Sum
  sin : Trigonometry
  sin{1,4..6} (4 alike) : Trigonometry  Operator=cos
  sin2 : Trigonometry
  sin3 : Trigonometry
  p : Outport  VectorParamsAs1DForOutWhenUnconnected=off
  q : Outport  Port=2  VectorParamsAs1DForOutWhenUnconnected=off
  r : Outport  Port=3  VectorParamsAs1DForOutWhenUnconnected=off
  wires:
  Phi dot/1 -> Sum/1
  Theta/1 -> sin4/1, sin6/1, sin/1
  sin/1 -> Product/1
  Psi dot/1 -> Product/2, Product2/3, Product4/1
  Product/1 -> Sum/2
  Sum/1 -> p/1
  Phi/1 -> sin1/1, sin2/1, sin3/1, sin5/1
  sin1/1 -> Product1/1
  Theta dot/1 -> Product1/2, Product3/1
  Product1/1 -> Sum1/1
  sin2/1 -> Product2/1
  sin4/1 -> Product2/2
  Product2/1 -> Sum1/2
  Sum1/1 -> q/1
  sin3/1 -> Product3/2
  sin5/1 -> Product4/2
  sin6/1 -> Product4/3
  Product3/1 -> Sum2/1
  Product4/1 -> Sum2/2
  Sum2/1 -> r/1

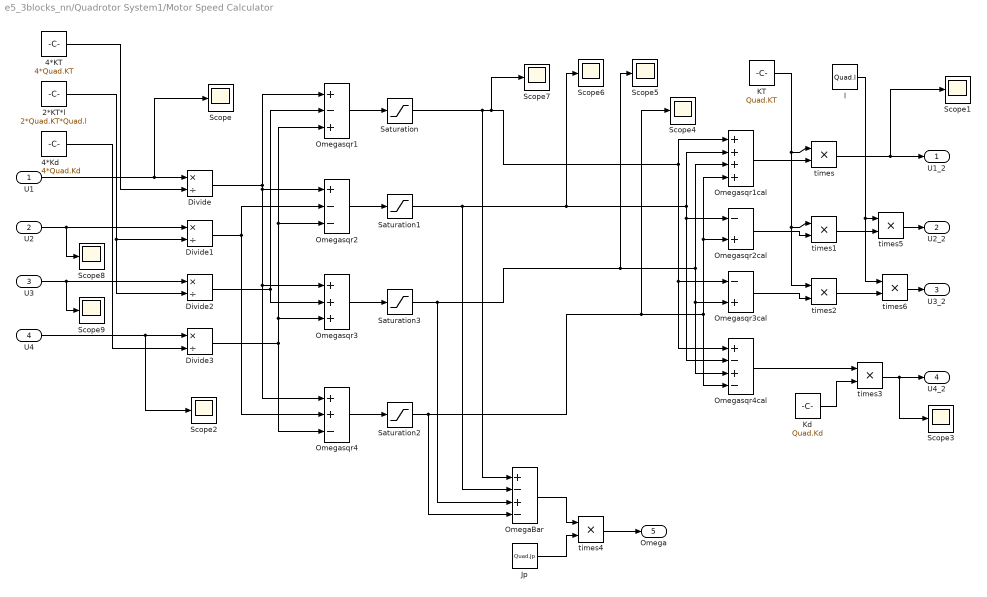
== system e5_3blocks_nn/Quadrotor System1/Motor Speed Calculator ==
  U1 : Inport
  U2 : Inport  Port=2
  U3 : Inport  Port=3
  U4 : Inport  Port=4
  2*KT*l : Constant  Value=2*Quad.KT*Quad.l
  4*KT : Constant  Value=4*Quad.KT
  4*Kd : Constant  Value=4*Quad.Kd
  Divide{,1..3} (4 alike) : Product  Inputs=*/
  Jp : Constant  Value=Quad.Jp
  KT : Constant  Value=Quad.KT
  Kd : Constant  Value=Quad.Kd
  OmegaBar : Sum  Inputs=+-+-
  Omegasqr1 : Sum  Inputs=+-+
  Omegasqr1cal : Sum  Inputs=++++
  Omegasqr2 : Sum  Inputs=+--
  Omegasqr2cal : Sum  Inputs=-+
  Omegasqr3 : Sum  Inputs=+++
  Omegasqr3cal : Sum  Inputs=-+
  Omegasqr4 : Sum  Inputs=++-
  Omegasqr4cal : Sum  Inputs=+-+-
  Saturation{,1..3} (4 alike) : Saturate  UpperLimit=Quad.max_motor_speed^2  LowerLimit=Quad.min_motor_speed^2  ZeroCross=off
  Scope{,1..9} (10 alike) : Scope
  l : Constant  Value=Quad.l
  times{,1..6} (7 alike) : Product  Inputs=**
  U1_2 : Outport  VectorParamsAs1DForOutWhenUnconnected=off
  U2_2 : Outport  Port=2  VectorParamsAs1DForOutWhenUnconnected=off
  U3_2 : Outport  Port=3  VectorParamsAs1DForOutWhenUnconnected=off
  U4_2 : Outport  Port=4  VectorParamsAs1DForOutWhenUnconnected=off
  Omega : Outport  Port=5  VectorParamsAs1DForOutWhenUnconnected=off
  wires:
  U1/1 -> Divide/1, Scope/1
  4*KT/1 -> Divide/2
  U2/1 -> Divide1/1, Scope8/1
  2*KT*l/1 -> Divide1/2, Divide2/2
  U3/1 -> Divide2/1, Scope9/1
  U4/1 -> Divide3/1, Scope2/1
  4*Kd/1 -> Divide3/2
  Divide/1 -> Omegasqr1/1, Omegasqr2/1, Omegasqr3/1, Omegasqr4/1
  Divide2/1 -> Omegasqr1/2, Omegasqr3/2
  Divide3/1 -> Omegasqr1/3, Omegasqr2/3, Omegasqr3/3, Omegasqr4/3
  Divide1/1 -> Omegasqr2/2, Omegasqr4/2
  OmegaBar/1 -> times4/1
  times4/1 -> Omega/1
  KT/1 -> times/1, times1/1, times2/1
  Omegasqr1cal/1 -> times/2
  Omegasqr2cal/1 -> times1/2
  Omegasqr3cal/1 -> times2/2
  Omegasqr4cal/1 -> times3/1
  Kd/1 -> times3/2
  times/1 -> U1_2/1, Scope1/1
  times3/1 -> U4_2/1, Scope3/1
  Jp/1 -> times4/2
  times5/1 -> U2_2/1
  times6/1 -> U3_2/1
  l/1 -> times5/1, times6/1
  times1/1 -> times5/2
  times2/1 -> times6/2
  Saturation/1 -> OmegaBar/1, Omegasqr1cal/1, Omegasqr3cal/1, Omegasqr4cal/1, Scope7/1
  Saturation2/1 -> OmegaBar/4, Omegasqr1cal/4, Omegasqr2cal/2, Omegasqr4cal/4, Scope4/1
  Saturation3/1 -> OmegaBar/3, Omegasqr1cal/3, Omegasqr3cal/2, Omegasqr4cal/3, Scope5/1
  Saturation1/1 -> OmegaBar/2, Omegasqr1cal/2, Omegasqr2cal/1, Omegasqr4cal/2, Scope6/1
  Omegasqr1/1 -> Saturation/1
  Omegasqr2/1 -> Saturation1/1
  Omegasqr3/1 -> Saturation3/1
  Omegasqr4/1 -> Saturation2/1

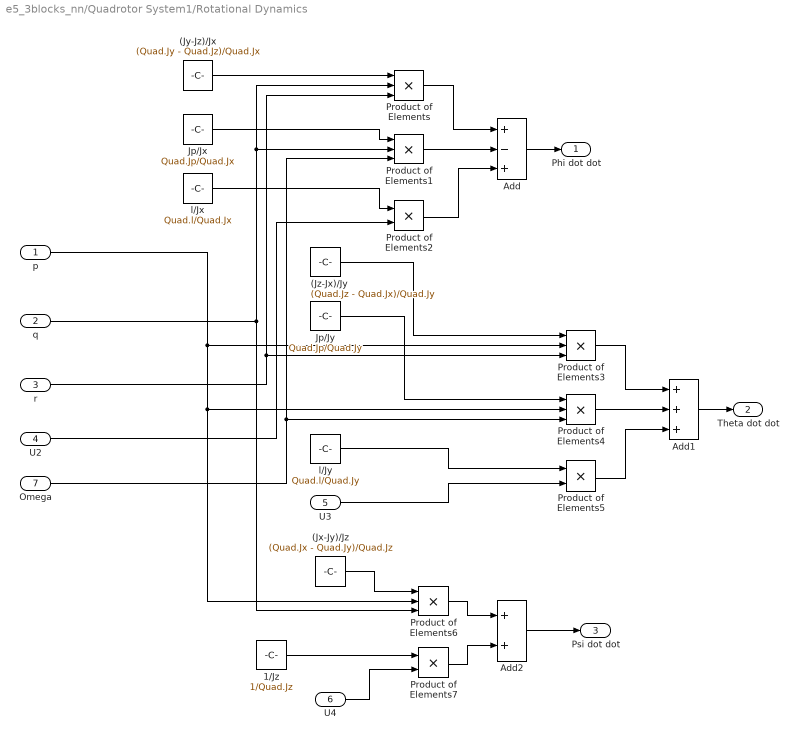
== system e5_3blocks_nn/Quadrotor System1/Rotational Dynamics ==
  p : Inport
  q : Inport  Port=2
  r : Inport  Port=3
  U2 : Inport  Port=4
  U3 : Inport  Port=5
  U4 : Inport  Port=6
  Omega : Inport  Port=7
  (Jx-Jy)/Jz : Constant  Value=(Quad.Jx - Quad.Jy)/Quad.Jz
  (Jy-Jz)/Jx : Constant  Value=(Quad.Jy - Quad.Jz)/Quad.Jx
  (Jz-Jx)/Jy : Constant  Value=(Quad.Jz - Quad.Jx)/Quad.Jy
  1/Jz : Constant  Value=1/Quad.Jz
  Add : Sum  Inputs=+-+
  Add1 : Sum  Inputs=+++
  Add2 : Sum
  Jp/Jx : Constant  Value=Quad.Jp/Quad.Jx
  Jp/Jy : Constant  Value=Quad.Jp/Quad.Jy
  Product of Elements{,1,3..4,6} (5 alike) : Product  Inputs=3
  Product of Elements2 : Product
  Product of Elements5 : Product
  Product of Elements7 : Product
  l/Jx : Constant  Value=Quad.l/Quad.Jx
  l/Jy : Constant  Value=Quad.l/Quad.Jy
  Phi dot dot : Outport  VectorParamsAs1DForOutWhenUnconnected=off
  Theta dot dot : Outport  Port=2  VectorParamsAs1DForOutWhenUnconnected=off
  Psi dot dot : Outport  Port=3  VectorParamsAs1DForOutWhenUnconnected=off
  wires:
  Product of Elements/1 -> Add/1
  Product of Elements1/1 -> Add/2
  Product of Elements2/1 -> Add/3
  Add/1 -> Phi dot dot/1
  (Jy-Jz)/Jx/1 -> Product of Elements/1
  q/1 -> Product of Elements/2, Product of Elements1/2, Product of Elements6/3
  r/1 -> Product of Elements/3, Product of Elements3/3
  Jp/Jx/1 -> Product of Elements1/1
  l/Jx/1 -> Product of Elements2/1
  U2/1 -> Product of Elements2/2
  Omega/1 -> Product of Elements1/3, Product of Elements4/3
  Product of Elements3/1 -> Add1/1
  Product of Elements4/1 -> Add1/2
  Product of Elements5/1 -> Add1/3
  Add1/1 -> Theta dot dot/1
  (Jz-Jx)/Jy/1 -> Product of Elements3/1
  Jp/Jy/1 -> Product of Elements4/1
  l/Jy/1 -> Product of Elements5/1
  U3/1 -> Product of Elements5/2
  p/1 -> Product of Elements3/2, Product of Elements4/2, Product of Elements6/2
  Product of Elements7/1 -> Add2/2
  Add2/1 -> Psi dot dot/1
  U4/1 -> Product of Elements7/2
  1/Jz/1 -> Product of Elements7/1
  (Jx-Jy)/Jz/1 -> Product of Elements6/1
  Product of Elements6/1 -> Add2/1

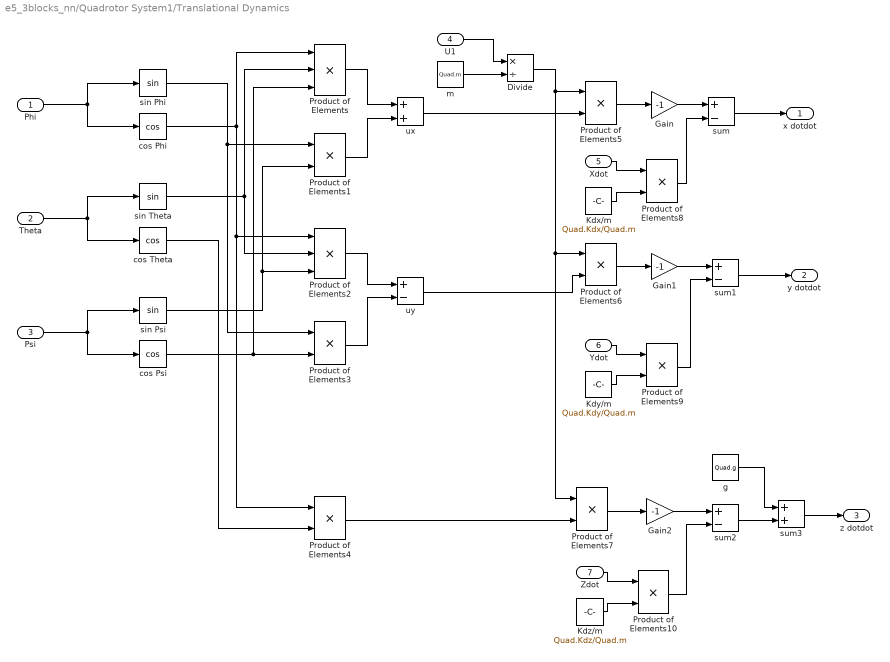
== system e5_3blocks_nn/Quadrotor System1/Translational Dynamics ==
  Phi : Inport
  Theta : Inport  Port=2
  Psi : Inport  Port=3
  U1 : Inport  Port=4
  Xdot : Inport  Port=5
  Ydot : Inport  Port=6
  Zdot : Inport  Port=7
  Divide : Product  Inputs=*/
  Gain : Gain  Gain=-1
  Gain1 : Gain  Gain=-1
  Gain2 : Gain  Gain=-1
  Kdx/m : Constant  Value=Quad.Kdx/Quad.m
  Kdy/m : Constant  Value=Quad.Kdy/Quad.m
  Kdz/m : Constant  Value=Quad.Kdz/Quad.m
  Product of Elements : Product  Inputs=3
  Product of Elements{1,3..10} (9 alike) : Product
  Product of Elements2 : Product  Inputs=3
  cos Phi : Trigonometry  Operator=cos
  cos Psi : Trigonometry  Operator=cos
  cos Theta : Trigonometry  Operator=cos
  g : Constant  Value=Quad.g
  m : Constant  Value=Quad.m
  sin Phi : Trigonometry
  sin Psi : Trigonometry
  sin Theta : Trigonometry
  sum : Sum  Inputs=+-
  sum1 : Sum  Inputs=+-
  sum2 : Sum  Inputs=+-
  sum3 : Sum
  ux : Sum
  uy : Sum  Inputs=+-
  x dotdot : Outport  VectorParamsAs1DForOutWhenUnconnected=off
  y dotdot : Outport  Port=2  VectorParamsAs1DForOutWhenUnconnected=off
  z dotdot : Outport  Port=3  VectorParamsAs1DForOutWhenUnconnected=off
  wires:
  Phi/1 -> sin Phi/1, cos Phi/1
  Theta/1 -> sin Theta/1, cos Theta/1
  Psi/1 -> sin Psi/1, cos Psi/1
  sin Theta/1 -> Product of Elements/2, Product of Elements2/2
  cos Psi/1 -> Product of Elements/3, Product of Elements3/2
  cos Phi/1 -> Product of Elements/1, Product of Elements2/1, Product of Elements4/1
  sin Phi/1 -> Product of Elements1/1, Product of Elements3/1
  sin Psi/1 -> Product of Elements1/2, Product of Elements2/3
  Product of Elements/1 -> ux/1
  Product of Elements1/1 -> ux/2
  ux/1 -> Product of Elements5/2
  Product of Elements2/1 -> uy/1
  Product of Elements3/1 -> uy/2
  uy/1 -> Product of Elements6/2
  cos Theta/1 -> Product of Elements4/2
  Product of Elements4/1 -> Product of Elements7/2
  U1/1 -> Divide/1
  m/1 -> Divide/2
  Divide/1 -> Product of Elements5/1, Product of Elements6/1, Product of Elements7/1
  sum3/1 -> z dotdot/1
  Product of Elements5/1 -> Gain/1
  Product of Elements6/1 -> Gain1/1
  Xdot/1 -> Product of Elements8/1
  Kdx/m/1 -> Product of Elements8/2
  Gain/1 -> sum/1
  Product of Elements8/1 -> sum/2
  sum/1 -> x dotdot/1
  Ydot/1 -> Product of Elements9/1
  Kdy/m/1 -> Product of Elements9/2
  Gain1/1 -> sum1/1
  Product of Elements9/1 -> sum1/2
  sum1/1 -> y dotdot/1
  Zdot/1 -> Product of Elements10/1
  Kdz/m/1 -> Product of Elements10/2
  Product of Elements7/1 -> Gain2/1
  g/1 -> sum3/1
  sum2/1 -> sum3/2
  Product of Elements10/1 -> sum2/2
  Gain2/1 -> sum2/1

== system e5_3blocks_nn/NN/Layer 1/Delays 1 ==
  "p{1}" : Inport  PortDimensions=15
      mask Display: e = 0.06;c1 = [120 230 180]/255;c2 = ([120 230 180]+0)/(256+128);c3 = ([120 230 180]+128)/(256+128);patch([0 1 1 0],[0 0 1 1],c1);patch([0 1 1 1-e 1-e 0+e],[0 0 1 1-e 0+e 0+e],c2);patch([0 0 1 1-e 0+e 0+e],[0 1 1 1-e 1-e 0+e],c3);plot([0 1 1 0 0],[0 0 1 1 0]);
  mux : Mux  Inputs=1
      mask Display: e = 0.06;c1 = [120 150 230]/255;c2 = ([120 150 230]+0)/383;c3 = ([120 150 230]+128)/383;patch([0 1 1 0],[0 0 1 1],c1);patch([0 1 1 1-e 1-e 0+e],[0 0 1 1-e 0+e 0+e],c2);patch([0 0 1 1-e 0+e 0+e],[0 1 1 1-e 1-e 0+e],c3);plot([0 1 1 0 0],[0 0 1 1 0]);disp('Mux')
  "pd{1,1}" : Outport
      mask Display: e = 0.06;c1 = [120 230 180]/255;c2 = ([120 230 180]+0)/(256+128);c3 = ([120 230 180]+128)/(256+128);patch([0 1 1 0],[0 0 1 1],c1);patch([0 1 1 1-e 1-e 0+e],[0 0 1 1-e 0+e 0+e],c2);patch([0 0 1 1-e 0+e 0+e],[0 1 1 1-e 1-e 0+e],c3);plot([0 1 1 0 0],[0 0 1 1 0]);
  wires:
  "p{1}"/1 -> mux/1
  mux/1 -> "pd{1,1}"/1
